simulink model "SUT_Test"  (Simulink 7.0)
settings: Solver=ode4  SolverMode=SingleTasking  StartTime=0.0  StopTime=252  FixedStep=0.01  RelTol=1e-3
InitFcn:
  | tempomat_para
StopFcn:
  | clear;
values from neighbouring files (symbols this model uses):
  A = 1.9    [tempomat_para.m]
  a_Fzg_max = 2    [tempomat_para.m]
  a_Fzg_min = -2    [tempomat_para.m]
  cw = 0.32    [tempomat_para.m]
  gang = [1 2 3 4]    [tempomat_para.m]
  gang_vec = [1 2 3 4]    [tempomat_para.m]
  i_anteil = 5    [tempomat_para.m]
  i_d = 3.42    [tempomat_para.m]
  i_g = [3.91 2.17 1.37 1.00]    [tempomat_para.m]
  lambda_gang = [1.3 1.25  1.17  1.05]    [tempomat_para.m]
  m_Fzg = 1400    [tempomat_para.m]
  M_mot_max = [130 149 163 170 168 166 162 158 150 139 123 80]    [tempomat_para.m]
  M_mot_min = [0 -40]    [tempomat_para.m]
  n_mot0 = 1000    [tempomat_para.m]
  n_mot_max = 1000:500:6500    [tempomat_para.m]
  n_mot_min = [1000 6500]    [tempomat_para.m]
  p_anteil = 100    [tempomat_para.m]
  r_dyn = 0.28    [tempomat_para.m]
  rho = 1.202    [tempomat_para.m]
  t_sch = 0.2    [tempomat_para.m]
  TI = [block '/TI']    [PSTI_callback.m]
  v_Fzg_ms0 = 0    [tempomat_para.m]
undefined symbols (not defined in the file or in its folder): Drossel_mat, getdatatypespecs
libraries: simulink x116, fzgbib x6
(part 10 of 11)

== system SUT_Test/Test Specification/R1 Speed Control step response/Maximum overshoot < 5 &  Steady state error < 5/Step response characteristics/Step response trigger/Active if signals constant for some specified time/Time since signal constant1 ==
  Signal : Inport  OutDataType=sfix(16)  OutScaling=2^0
  Clock : Clock
      settings: Decimation=10
  Detect constant : Subsystem  TreatAsAtomicUnit=on  mask(Feature extraction block){RT=0.0001}
      mask prompts: RT "Relative tolerance in %"
      mask help: Detect if the signal value is constant (using the last two signal values) allowing for a user-defined relative deviation
      mask CallbackString:
      | if or( (str2double(get_param(gcb,'RT')) < 0), (str2double(get_param(gcb,'RT')) > 100))
      |     error(['Relative tolerance value (' get_param(gcb,'RT') ') out of range. Please give a value between 0 and 100.']);
      | else
      |     set_param([gcb '/Relative tolerance/Relative Tolerance'],'Value',get_param(gcb,'RT'));
      | end
  Logical Operator : Logic  Operator=NAND  AllPortsSameDT=off  OutDataTypeMode=boolean
  Logical Operator1 : Logic  Operator=NOT  AllPortsSameDT=off  OutDataTypeMode=boolean
  Memory : Memory  Orientation=left
  Memory1 : Memory
  Subtract : Sum  Inputs=-+  OutDataType=sfix(16)  OutScaling=2^-10
  Switch : Switch  Criteria=u2 > Threshold
  Trigger : Outport  OutDataType=sfix(16)  OutScaling=2^0
  Feature : Outport  Port=2  OutDataType=sfix(16)  OutScaling=2^0
  wires:
  Logical Operator/1 -> Switch/2
  Logical Operator1/1 -> Logical Operator/2
  Memory1/1 -> Logical Operator1/1
  Memory/1 -> Switch/1
  Switch/1 -> Memory/1, Subtract/1
  Clock/1 -> Switch/3, Subtract/2
  Subtract/1 -> Feature/1
  Detect constant/1(Constant) -> Memory1/1, Logical Operator/1, Trigger/1
  Signal/1 -> Detect constant/1(Signal)

== system SUT_Test/Test Specification/R2 Speed Control velocity restoration time after simple  acceleration/deceleration/CC active + no target & Speed Control active & step of V_Des = |1|  with time periods >= 7s/Step with step size=|1|  and time periods >= 6s detection/Step detection/Active if signals constant for some specified time/Time since signal constant1 ==
  Signal : Inport  OutDataType=sfix(16)  OutScaling=2^0
  Clock : Clock
      settings: Decimation=10
  Detect constant : Subsystem  TreatAsAtomicUnit=on  mask(Feature extraction block){RT=0.0001}
      mask prompts: RT "Relative tolerance in %"
      mask help: Detect if the signal value is constant (using the last two signal values) allowing for a user-defined relative deviation
      mask CallbackString:
      | if or( (str2double(get_param(gcb,'RT')) < 0), (str2double(get_param(gcb,'RT')) > 100))
      |     error(['Relative tolerance value (' get_param(gcb,'RT') ') out of range. Please give a value between 0 and 100.']);
      | else
      |     set_param([gcb '/Relative tolerance/Relative Tolerance'],'Value',get_param(gcb,'RT'));
      | end
  Logical Operator : Logic  Operator=NAND  AllPortsSameDT=off  OutDataTypeMode=boolean
  Logical Operator1 : Logic  Operator=NOT  AllPortsSameDT=off  OutDataTypeMode=boolean
  Memory : Memory  Orientation=left
  Memory1 : Memory
  Subtract : Sum  Inputs=-+  OutDataType=sfix(16)  OutScaling=2^-10
  Switch : Switch  Criteria=u2 > Threshold
  Trigger : Outport  OutDataType=sfix(16)  OutScaling=2^0
  Feature : Outport  Port=2  OutDataType=sfix(16)  OutScaling=2^0
  wires:
  Logical Operator/1 -> Switch/2
  Logical Operator1/1 -> Logical Operator/2
  Memory1/1 -> Logical Operator1/1
  Memory/1 -> Switch/1
  Switch/1 -> Memory/1, Subtract/1
  Clock/1 -> Switch/3, Subtract/2
  Subtract/1 -> Feature/1
  Detect constant/1(Constant) -> Memory1/1, Logical Operator/1, Trigger/1
  Signal/1 -> Detect constant/1(Signal)

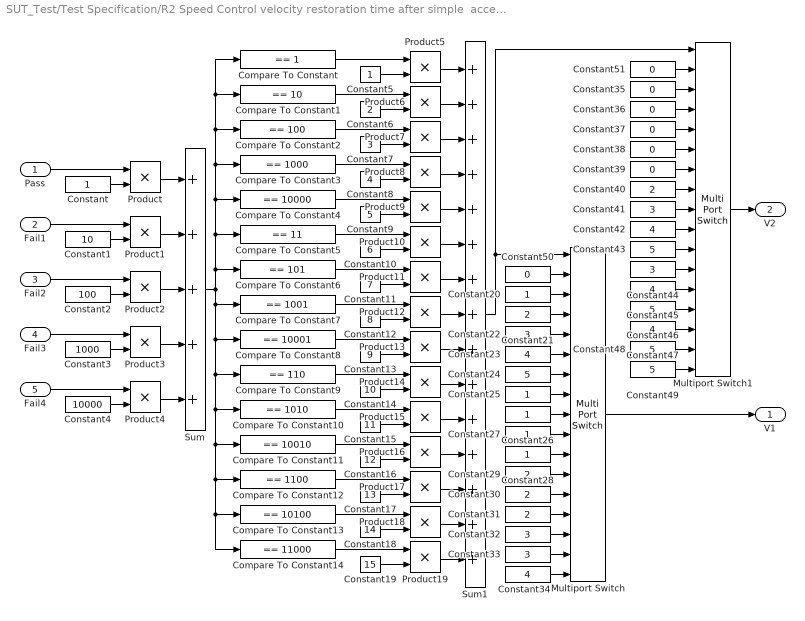
== system SUT_Test/Test Specification/R2 Speed Control velocity restoration time after simple  acceleration/deceleration/after (6 seconds)  |V_Des-V_Vhcl <= 1.4|/PAS1/none - pass - fail/Arbitration/Verdict identification ==
  Pass : Inport  OutDataType=sfix(16)  OutScaling=2^0
  Fail1 : Inport  Port=2  OutDataType=sfix(16)  OutScaling=2^0
  Fail2 : Inport  Port=3  OutDataType=sfix(16)  OutScaling=2^0
  Fail3 : Inport  Port=4  OutDataType=sfix(16)  OutScaling=2^0
  Fail4 : Inport  Port=5  OutDataType=sfix(16)  OutScaling=2^0
  Compare To Constant : simulink/Logic and Bit Operations/Compare To Constant  SystemSampleTime=-1  relop===  const=1  LogicOutDataTypeMode=uint8  ZeroCross=off
  Compare To Constant1 : simulink/Logic and Bit Operations/Compare To Constant  SystemSampleTime=-1  relop===  const=10  LogicOutDataTypeMode=uint8  ZeroCross=off
  Compare To Constant10 : simulink/Logic and Bit Operations/Compare To Constant  SystemSampleTime=-1  relop===  const=1010  LogicOutDataTypeMode=uint8  ZeroCross=off
  Compare To Constant11 : simulink/Logic and Bit Operations/Compare To Constant  SystemSampleTime=-1  relop===  const=10010  LogicOutDataTypeMode=uint8  ZeroCross=off
  Compare To Constant12 : simulink/Logic and Bit Operations/Compare To Constant  SystemSampleTime=-1  relop===  const=1100  LogicOutDataTypeMode=uint8  ZeroCross=off
  Compare To Constant13 : simulink/Logic and Bit Operations/Compare To Constant  SystemSampleTime=-1  relop===  const=10100  LogicOutDataTypeMode=uint8  ZeroCross=off
  Compare To Constant14 : simulink/Logic and Bit Operations/Compare To Constant  SystemSampleTime=-1  relop===  const=11000  LogicOutDataTypeMode=uint8  ZeroCross=off
  Compare To Constant2 : simulink/Logic and Bit Operations/Compare To Constant  SystemSampleTime=-1  relop===  const=100  LogicOutDataTypeMode=uint8  ZeroCross=off
  Compare To Constant3 : simulink/Logic and Bit Operations/Compare To Constant  SystemSampleTime=-1  relop===  const=1000  LogicOutDataTypeMode=uint8  ZeroCross=off
  Compare To Constant4 : simulink/Logic and Bit Operations/Compare To Constant  SystemSampleTime=-1  relop===  const=10000  LogicOutDataTypeMode=uint8  ZeroCross=off
  Compare To Constant5 : simulink/Logic and Bit Operations/Compare To Constant  SystemSampleTime=-1  relop===  const=11  LogicOutDataTypeMode=uint8  ZeroCross=off
  Compare To Constant6 : simulink/Logic and Bit Operations/Compare To Constant  SystemSampleTime=-1  relop===  const=101  LogicOutDataTypeMode=uint8  ZeroCross=off
  Compare To Constant7 : simulink/Logic and Bit Operations/Compare To Constant  SystemSampleTime=-1  relop===  const=1001  LogicOutDataTypeMode=uint8  ZeroCross=off
  Compare To Constant8 : simulink/Logic and Bit Operations/Compare To Constant  SystemSampleTime=-1  relop===  const=10001  LogicOutDataTypeMode=uint8  ZeroCross=off
  Compare To Constant9 : simulink/Logic and Bit Operations/Compare To Constant  SystemSampleTime=-1  relop===  const=110  LogicOutDataTypeMode=uint8  ZeroCross=off
  Constant{,5,20,25..28} (7 alike) : Constant  OutDataType=sfix(16)  OutScaling=2^0
  Constant1 : Constant  Value=10  OutDataType=sfix(16)  OutScaling=2^0
  Constant10 : Constant  Value=6  OutDataType=sfix(16)  OutScaling=2^0
  Constant11 : Constant  Value=7  OutDataType=sfix(16)  OutScaling=2^0
  Constant12 : Constant  Value=8  OutDataType=sfix(16)  OutScaling=2^0
  Constant13 : Constant  Value=9  OutDataType=sfix(16)  OutScaling=2^0
  Constant14 : Constant  Value=10  OutDataType=sfix(16)  OutScaling=2^0
  Constant15 : Constant  Value=11  OutDataType=sfix(16)  OutScaling=2^0
  Constant16 : Constant  Value=12  OutDataType=sfix(16)  OutScaling=2^0
  Constant17 : Constant  Value=13  OutDataType=sfix(16)  OutScaling=2^0
  Constant18 : Constant  Value=14  OutDataType=sfix(16)  OutScaling=2^0
  Constant19 : Constant  Value=15  OutDataType=sfix(16)  OutScaling=2^0
  Constant2 : Constant  Value=100  OutDataType=sfix(16)  OutScaling=2^0
  Constant{6,21,29..31,40} (6 alike) : Constant  Value=2  OutDataType=sfix(16)  OutScaling=2^0
  Constant{7,22,32..33,41,44} (6 alike) : Constant  Value=3  OutDataType=sfix(16)  OutScaling=2^0
  Constant{8,23,34,42,45,47} (6 alike) : Constant  Value=4  OutDataType=sfix(16)  OutScaling=2^0
  Constant{9,24,43,46,48..49} (6 alike) : Constant  Value=5  OutDataType=sfix(16)  OutScaling=2^0
  Constant3 : Constant  Value=1000  OutDataType=sfix(16)  OutScaling=2^0
  Constant{35..39,50..51} (7 alike) : Constant  Value=0  OutDataType=sfix(16)  OutScaling=2^0
  Constant4 : Constant  Value=10000  OutDataType=sfix(16)  OutScaling=2^0
  Multiport Switch : MultiPortSwitch  Inputs=16  zeroidx=on
  Multiport Switch1 : MultiPortSwitch  Inputs=16  zeroidx=on
  Product{,1..19} (20 alike) : Product  OutDataType=sfix(16)  OutScaling=2^0  RndMeth=Zero
  Sum : Sum  Inputs=+++++  OutDataType=sfix(16)  OutScaling=2^0
  Sum1 : Sum  Inputs=+++++++++++++++  OutDataType=sfix(16)  OutScaling=2^0
  V1 : Outport  OutDataType=sfix(16)  OutScaling=2^0
  V2 : Outport  Port=2  OutDataType=sfix(16)  OutScaling=2^0
  wires:
  Constant51/1 -> Multiport Switch1/2
  Constant34/1 -> Multiport Switch/17
  Constant33/1 -> Multiport Switch/16
  Constant32/1 -> Multiport Switch/15
  Constant31/1 -> Multiport Switch/14
  Constant30/1 -> Multiport Switch/13
  Constant29/1 -> Multiport Switch/12
  Constant28/1 -> Multiport Switch/11
  Constant27/1 -> Multiport Switch/10
  Constant26/1 -> Multiport Switch/9
  Constant25/1 -> Multiport Switch/8
  Constant24/1 -> Multiport Switch/7
  Constant23/1 -> Multiport Switch/6
  Constant22/1 -> Multiport Switch/5
  Constant21/1 -> Multiport Switch/4
  Constant20/1 -> Multiport Switch/3
  Constant50/1 -> Multiport Switch/2
  Product19/1 -> Sum1/15
  Product18/1 -> Sum1/14
  Product17/1 -> Sum1/13
  Product16/1 -> Sum1/12
  Product15/1 -> Sum1/11
  Product14/1 -> Sum1/10
  Product13/1 -> Sum1/9
  Product12/1 -> Sum1/8
  Product11/1 -> Sum1/7
  Product10/1 -> Sum1/6
  Product9/1 -> Sum1/5
  Product8/1 -> Sum1/4
  Product7/1 -> Sum1/3
  Product6/1 -> Sum1/2
  Product5/1 -> Sum1/1
  Multiport Switch1/1 -> V2/1
  Constant49/1 -> Multiport Switch1/17
  Constant48/1 -> Multiport Switch1/16
  Constant47/1 -> Multiport Switch1/15
  Constant46/1 -> Multiport Switch1/14
  Constant45/1 -> Multiport Switch1/13
  Constant44/1 -> Multiport Switch1/12
  Constant43/1 -> Multiport Switch1/11
  Constant42/1 -> Multiport Switch1/10
  Constant41/1 -> Multiport Switch1/9
  Constant40/1 -> Multiport Switch1/8
  Constant39/1 -> Multiport Switch1/7
  Constant38/1 -> Multiport Switch1/6
  Constant37/1 -> Multiport Switch1/5
  Constant36/1 -> Multiport Switch1/4
  Constant35/1 -> Multiport Switch1/3
  Sum1/1 -> Multiport Switch1/1, Multiport Switch/1
  Multiport Switch/1 -> V1/1
  Sum/1 -> Compare To Constant7/1, Compare To Constant13/1, Compare To Constant14/1, Compare To Constant12/1, Compare To Constant11/1, Compare To Constant10/1, Compare To Constant9/1, Compare To Constant8/1, Compare To Constant/1, Compare To Constant1/1, Compare To Constant2/1, Compare To Constant3/1, Compare To Constant4/1, Compare To Constant5/1, Compare To Constant6/1
  Compare To Constant14/1 -> Product19/1
  Constant19/1 -> Product19/2
  Compare To Constant13/1 -> Product18/1
  Constant18/1 -> Product18/2
  Compare To Constant12/1 -> Product17/1
  Constant17/1 -> Product17/2
  Compare To Constant11/1 -> Product16/1
  Constant16/1 -> Product16/2
  Compare To Constant10/1 -> Product15/1
  Constant15/1 -> Product15/2
  Compare To Constant9/1 -> Product14/1
  Constant14/1 -> Product14/2
  Compare To Constant8/1 -> Product13/1
  Constant13/1 -> Product13/2
  Compare To Constant7/1 -> Product12/1
  Constant12/1 -> Product12/2
  Compare To Constant6/1 -> Product11/1
  Constant11/1 -> Product11/2
  Compare To Constant5/1 -> Product10/1
  Constant10/1 -> Product10/2
  Compare To Constant4/1 -> Product9/1
  Constant9/1 -> Product9/2
  Compare To Constant3/1 -> Product8/1
  Compare To Constant2/1 -> Product7/1
  Constant8/1 -> Product8/2
  Constant7/1 -> Product7/2
  Compare To Constant1/1 -> Product6/1
  Constant6/1 -> Product6/2
  Constant5/1 -> Product5/2
  Compare To Constant/1 -> Product5/1
  Product4/1 -> Sum/5
  Product3/1 -> Sum/4
  Product2/1 -> Sum/3
  Product1/1 -> Sum/2
  Product/1 -> Sum/1
  Constant/1 -> Product/2
  Constant1/1 -> Product1/2
  Constant2/1 -> Product2/2
  Constant4/1 -> Product4/2
  Constant3/1 -> Product3/2
  Fail4/1 -> Product4/1
  Fail3/1 -> Product3/1
  Fail2/1 -> Product2/1
  Fail1/1 -> Product1/1
  Pass/1 -> Product/1

== system SUT_Test/Test Specification/R2 Speed Control velocity restoration time after simple  acceleration/deceleration/after (6 seconds)  |V_Des-V_Vhcl <= 1.4|/PAS1/none - pass - fail/Arbitration/Verdict selection ==
  V1 : Inport  OutDataType=sfix(16)  OutScaling=2^0
  V2 : Inport  Port=2  OutDataType=sfix(16)  OutScaling=2^0
  Delay P F1 F3 : Inport  Port=3  OutDataType=sfix(16)  OutScaling=2^0
  Delay F2 : Inport  Port=4  OutDataType=sfix(16)  OutScaling=2^0
  Delay F4 : Inport  Port=5  OutDataType=sfix(16)  OutScaling=2^0
  Max delay : Inport  Port=6  OutDataType=sfix(16)  OutScaling=2^0
  Compare To Zero1 : simulink/Logic and Bit Operations/Compare To Zero  SystemSampleTime=-1  relop=~=  LogicOutDataTypeMode=boolean  ZeroCross=off
  Constant{2..4,39} (4 alike) : Constant  Value=0  OutDataType=sfix(16)  OutScaling=2^0
  Constant35 : Constant  OutDataType=sfix(16)  OutScaling=2^0
  Constant40 : Constant  Value=2  OutDataType=sfix(16)  OutScaling=2^0
  Memory : Memory
  Memory1 : Memory
  Multiport Switch1 : MultiPortSwitch  Inputs=6  zeroidx=on
  Multiport Switch2 : MultiPortSwitch  Inputs=6  zeroidx=on
  Multiport Switch4 : MultiPortSwitch  Inputs=6  zeroidx=on
  Sum : Sum  OutDataType=sfix(16)  OutScaling=2^0
  Switch : Switch  Criteria=u2 ~= 0
  Switch1 : Switch  Criteria=u2 ~= 0
  Switch2 : Switch  Criteria=u2 ~= 0
  Unit : Constant  OutDataType=sfix(16)  OutScaling=2^0
  Verdict : Outport  OutDataType=sfix(16)  OutScaling=2^0
  Delay : Outport  Port=2  OutDataType=sfix(16)  OutScaling=2^0
  wires:
  Switch2/1 -> Multiport Switch4/1, Memory/1
  Unit/1 -> Sum/1
  Memory1/1 -> Sum/2
  Sum/1 -> Switch1/1
  Multiport Switch4/1 -> Memory1/1
  Multiport Switch2/1 -> Switch1/3
  Switch1/1 -> Delay/1
  Switch/1 -> Multiport Switch1/1
  Compare To Zero1/1 -> Switch2/2, Switch1/2, Switch/2
  Memory/1 -> Switch/1, Compare To Zero1/1
  Delay F4/1 -> Multiport Switch4/7, Multiport Switch2/7
  Delay F2/1 -> Multiport Switch4/5, Multiport Switch2/5
  Delay P F1 F3/1 -> Multiport Switch4/3, Multiport Switch4/4, Multiport Switch4/6, Multiport Switch2/4, Multiport Switch2/6, Multiport Switch2/3
  Max delay/1 -> Multiport Switch4/2, Multiport Switch2/2
  V1/1 -> Switch2/1, Switch/3, Multiport Switch2/1
  V2/1 -> Switch2/3
  Constant40/1 -> Multiport Switch1/2
  Constant35/1 -> Multiport Switch1/3
  Constant4/1 -> Multiport Switch1/4
  Constant3/1 -> Multiport Switch1/5
  Constant2/1 -> Multiport Switch1/6
  Constant39/1 -> Multiport Switch1/7
  Multiport Switch1/1 -> Verdict/1

== system SUT_Test/Test Specification/R2 Speed Control velocity restoration time after simple  acceleration/deceleration/after (6 seconds)  |V_Des-V_Vhcl <= 1.4|/PAS1/none - pass - fail/Compute delay/Hold1 ==
  " " : Inport  OutDataType=sfix(16)  OutScaling=2^0
  "    " : Inport  Port=2  OutDataType=sfix(16)  OutScaling=2^0
  Memory : Memory  Orientation=left
  Switch : Switch  Criteria=u2 ~= 0
  "  " : Outport  OutDataType=sfix(16)  OutScaling=2^0
  wires:
  " "/1 -> Switch/2
  "    "/1 -> Switch/1
  Switch/1 -> "  "/1, Memory/1
  Memory/1 -> Switch/3

== system SUT_Test/Test Specification/R2 Speed Control velocity restoration time after simple  acceleration/deceleration/after (6 seconds)  |V_Des-V_Vhcl <= 1.4|/PAS1/none - pass - fail/Compute delay1/Hold1 ==
  " " : Inport  OutDataType=sfix(16)  OutScaling=2^0
  "    " : Inport  Port=2  OutDataType=sfix(16)  OutScaling=2^0
  Memory : Memory  Orientation=left
  Switch : Switch  Criteria=u2 ~= 0
  "  " : Outport  OutDataType=sfix(16)  OutScaling=2^0
  wires:
  " "/1 -> Switch/2
  "    "/1 -> Switch/1
  Switch/1 -> "  "/1, Memory/1
  Memory/1 -> Switch/3

== system SUT_Test/Test Specification/R2 Speed Control velocity restoration time after simple  acceleration/deceleration/after (6 seconds)  |V_Des-V_Vhcl <= 1.4|/PAS1/none - pass - fail/Compute delay2/Hold1 ==
  " " : Inport  OutDataType=sfix(16)  OutScaling=2^0
  "    " : Inport  Port=2  OutDataType=sfix(16)  OutScaling=2^0
  Memory : Memory  Orientation=left
  Switch : Switch  Criteria=u2 ~= 0
  "  " : Outport  OutDataType=sfix(16)  OutScaling=2^0
  wires:
  Memory/1 -> Switch/3
  Switch/1 -> Memory/1, "  "/1
  "    "/1 -> Switch/1
  " "/1 -> Switch/2

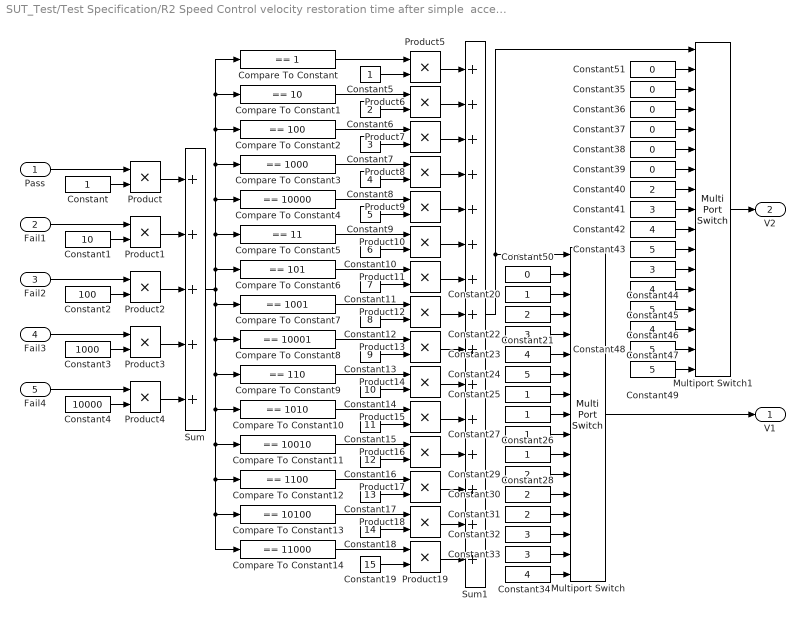
== system SUT_Test/Test Specification/R2 Speed Control velocity restoration time after simple  acceleration/deceleration/after (6 seconds)  |V_Des-V_Vhcl <= 1.4|/PAS2/none - pass - fail/Arbitration/Verdict identification ==
  Pass : Inport  OutDataType=sfix(16)  OutScaling=2^0
  Fail1 : Inport  Port=2  OutDataType=sfix(16)  OutScaling=2^0
  Fail2 : Inport  Port=3  OutDataType=sfix(16)  OutScaling=2^0
  Fail3 : Inport  Port=4  OutDataType=sfix(16)  OutScaling=2^0
  Fail4 : Inport  Port=5  OutDataType=sfix(16)  OutScaling=2^0
  Compare To Constant : simulink/Logic and Bit Operations/Compare To Constant  SystemSampleTime=-1  relop===  const=1  LogicOutDataTypeMode=uint8  ZeroCross=off
  Compare To Constant1 : simulink/Logic and Bit Operations/Compare To Constant  SystemSampleTime=-1  relop===  const=10  LogicOutDataTypeMode=uint8  ZeroCross=off
  Compare To Constant10 : simulink/Logic and Bit Operations/Compare To Constant  SystemSampleTime=-1  relop===  const=1010  LogicOutDataTypeMode=uint8  ZeroCross=off
  Compare To Constant11 : simulink/Logic and Bit Operations/Compare To Constant  SystemSampleTime=-1  relop===  const=10010  LogicOutDataTypeMode=uint8  ZeroCross=off
  Compare To Constant12 : simulink/Logic and Bit Operations/Compare To Constant  SystemSampleTime=-1  relop===  const=1100  LogicOutDataTypeMode=uint8  ZeroCross=off
  Compare To Constant13 : simulink/Logic and Bit Operations/Compare To Constant  SystemSampleTime=-1  relop===  const=10100  LogicOutDataTypeMode=uint8  ZeroCross=off
  Compare To Constant14 : simulink/Logic and Bit Operations/Compare To Constant  SystemSampleTime=-1  relop===  const=11000  LogicOutDataTypeMode=uint8  ZeroCross=off
  Compare To Constant2 : simulink/Logic and Bit Operations/Compare To Constant  SystemSampleTime=-1  relop===  const=100  LogicOutDataTypeMode=uint8  ZeroCross=off
  Compare To Constant3 : simulink/Logic and Bit Operations/Compare To Constant  SystemSampleTime=-1  relop===  const=1000  LogicOutDataTypeMode=uint8  ZeroCross=off
  Compare To Constant4 : simulink/Logic and Bit Operations/Compare To Constant  SystemSampleTime=-1  relop===  const=10000  LogicOutDataTypeMode=uint8  ZeroCross=off
  Compare To Constant5 : simulink/Logic and Bit Operations/Compare To Constant  SystemSampleTime=-1  relop===  const=11  LogicOutDataTypeMode=uint8  ZeroCross=off
  Compare To Constant6 : simulink/Logic and Bit Operations/Compare To Constant  SystemSampleTime=-1  relop===  const=101  LogicOutDataTypeMode=uint8  ZeroCross=off
  Compare To Constant7 : simulink/Logic and Bit Operations/Compare To Constant  SystemSampleTime=-1  relop===  const=1001  LogicOutDataTypeMode=uint8  ZeroCross=off
  Compare To Constant8 : simulink/Logic and Bit Operations/Compare To Constant  SystemSampleTime=-1  relop===  const=10001  LogicOutDataTypeMode=uint8  ZeroCross=off
  Compare To Constant9 : simulink/Logic and Bit Operations/Compare To Constant  SystemSampleTime=-1  relop===  const=110  LogicOutDataTypeMode=uint8  ZeroCross=off
  Constant{,5,20,25..28} (7 alike) : Constant  OutDataType=sfix(16)  OutScaling=2^0
  Constant1 : Constant  Value=10  OutDataType=sfix(16)  OutScaling=2^0
  Constant10 : Constant  Value=6  OutDataType=sfix(16)  OutScaling=2^0
  Constant11 : Constant  Value=7  OutDataType=sfix(16)  OutScaling=2^0
  Constant12 : Constant  Value=8  OutDataType=sfix(16)  OutScaling=2^0
  Constant13 : Constant  Value=9  OutDataType=sfix(16)  OutScaling=2^0
  Constant14 : Constant  Value=10  OutDataType=sfix(16)  OutScaling=2^0
  Constant15 : Constant  Value=11  OutDataType=sfix(16)  OutScaling=2^0
  Constant16 : Constant  Value=12  OutDataType=sfix(16)  OutScaling=2^0
  Constant17 : Constant  Value=13  OutDataType=sfix(16)  OutScaling=2^0
  Constant18 : Constant  Value=14  OutDataType=sfix(16)  OutScaling=2^0
  Constant19 : Constant  Value=15  OutDataType=sfix(16)  OutScaling=2^0
  Constant2 : Constant  Value=100  OutDataType=sfix(16)  OutScaling=2^0
  Constant{6,21,29..31,40} (6 alike) : Constant  Value=2  OutDataType=sfix(16)  OutScaling=2^0
  Constant{7,22,32..33,41,44} (6 alike) : Constant  Value=3  OutDataType=sfix(16)  OutScaling=2^0
  Constant{8,23,34,42,45,47} (6 alike) : Constant  Value=4  OutDataType=sfix(16)  OutScaling=2^0
  Constant{9,24,43,46,48..49} (6 alike) : Constant  Value=5  OutDataType=sfix(16)  OutScaling=2^0
  Constant3 : Constant  Value=1000  OutDataType=sfix(16)  OutScaling=2^0
  Constant{35..39,50..51} (7 alike) : Constant  Value=0  OutDataType=sfix(16)  OutScaling=2^0
  Constant4 : Constant  Value=10000  OutDataType=sfix(16)  OutScaling=2^0
  Multiport Switch : MultiPortSwitch  Inputs=16  zeroidx=on
  Multiport Switch1 : MultiPortSwitch  Inputs=16  zeroidx=on
  Product{,1..19} (20 alike) : Product  OutDataType=sfix(16)  OutScaling=2^0  RndMeth=Zero
  Sum : Sum  Inputs=+++++  OutDataType=sfix(16)  OutScaling=2^0
  Sum1 : Sum  Inputs=+++++++++++++++  OutDataType=sfix(16)  OutScaling=2^0
  V1 : Outport  OutDataType=sfix(16)  OutScaling=2^0
  V2 : Outport  Port=2  OutDataType=sfix(16)  OutScaling=2^0
  wires:
  Constant51/1 -> Multiport Switch1/2
  Constant34/1 -> Multiport Switch/17
  Constant33/1 -> Multiport Switch/16
  Constant32/1 -> Multiport Switch/15
  Constant31/1 -> Multiport Switch/14
  Constant30/1 -> Multiport Switch/13
  Constant29/1 -> Multiport Switch/12
  Constant28/1 -> Multiport Switch/11
  Constant27/1 -> Multiport Switch/10
  Constant26/1 -> Multiport Switch/9
  Constant25/1 -> Multiport Switch/8
  Constant24/1 -> Multiport Switch/7
  Constant23/1 -> Multiport Switch/6
  Constant22/1 -> Multiport Switch/5
  Constant21/1 -> Multiport Switch/4
  Constant20/1 -> Multiport Switch/3
  Constant50/1 -> Multiport Switch/2
  Product19/1 -> Sum1/15
  Product18/1 -> Sum1/14
  Product17/1 -> Sum1/13
  Product16/1 -> Sum1/12
  Product15/1 -> Sum1/11
  Product14/1 -> Sum1/10
  Product13/1 -> Sum1/9
  Product12/1 -> Sum1/8
  Product11/1 -> Sum1/7
  Product10/1 -> Sum1/6
  Product9/1 -> Sum1/5
  Product8/1 -> Sum1/4
  Product7/1 -> Sum1/3
  Product6/1 -> Sum1/2
  Product5/1 -> Sum1/1
  Multiport Switch1/1 -> V2/1
  Constant49/1 -> Multiport Switch1/17
  Constant48/1 -> Multiport Switch1/16
  Constant47/1 -> Multiport Switch1/15
  Constant46/1 -> Multiport Switch1/14
  Constant45/1 -> Multiport Switch1/13
  Constant44/1 -> Multiport Switch1/12
  Constant43/1 -> Multiport Switch1/11
  Constant42/1 -> Multiport Switch1/10
  Constant41/1 -> Multiport Switch1/9
  Constant40/1 -> Multiport Switch1/8
  Constant39/1 -> Multiport Switch1/7
  Constant38/1 -> Multiport Switch1/6
  Constant37/1 -> Multiport Switch1/5
  Constant36/1 -> Multiport Switch1/4
  Constant35/1 -> Multiport Switch1/3
  Sum1/1 -> Multiport Switch1/1, Multiport Switch/1
  Multiport Switch/1 -> V1/1
  Sum/1 -> Compare To Constant7/1, Compare To Constant13/1, Compare To Constant14/1, Compare To Constant12/1, Compare To Constant11/1, Compare To Constant10/1, Compare To Constant9/1, Compare To Constant8/1, Compare To Constant/1, Compare To Constant1/1, Compare To Constant2/1, Compare To Constant3/1, Compare To Constant4/1, Compare To Constant5/1, Compare To Constant6/1
  Compare To Constant14/1 -> Product19/1
  Constant19/1 -> Product19/2
  Compare To Constant13/1 -> Product18/1
  Constant18/1 -> Product18/2
  Compare To Constant12/1 -> Product17/1
  Constant17/1 -> Product17/2
  Compare To Constant11/1 -> Product16/1
  Constant16/1 -> Product16/2
  Compare To Constant10/1 -> Product15/1
  Constant15/1 -> Product15/2
  Compare To Constant9/1 -> Product14/1
  Constant14/1 -> Product14/2
  Compare To Constant8/1 -> Product13/1
  Constant13/1 -> Product13/2
  Compare To Constant7/1 -> Product12/1
  Constant12/1 -> Product12/2
  Compare To Constant6/1 -> Product11/1
  Constant11/1 -> Product11/2
  Compare To Constant5/1 -> Product10/1
  Constant10/1 -> Product10/2
  Compare To Constant4/1 -> Product9/1
  Constant9/1 -> Product9/2
  Compare To Constant3/1 -> Product8/1
  Compare To Constant2/1 -> Product7/1
  Constant8/1 -> Product8/2
  Constant7/1 -> Product7/2
  Compare To Constant1/1 -> Product6/1
  Constant6/1 -> Product6/2
  Constant5/1 -> Product5/2
  Compare To Constant/1 -> Product5/1
  Product4/1 -> Sum/5
  Product3/1 -> Sum/4
  Product2/1 -> Sum/3
  Product1/1 -> Sum/2
  Product/1 -> Sum/1
  Constant/1 -> Product/2
  Constant1/1 -> Product1/2
  Constant2/1 -> Product2/2
  Constant4/1 -> Product4/2
  Constant3/1 -> Product3/2
  Fail4/1 -> Product4/1
  Fail3/1 -> Product3/1
  Fail2/1 -> Product2/1
  Fail1/1 -> Product1/1
  Pass/1 -> Product/1

== system SUT_Test/Test Specification/R2 Speed Control velocity restoration time after simple  acceleration/deceleration/after (6 seconds)  |V_Des-V_Vhcl <= 1.4|/PAS2/none - pass - fail/Arbitration/Verdict selection ==
  V1 : Inport  OutDataType=sfix(16)  OutScaling=2^0
  V2 : Inport  Port=2  OutDataType=sfix(16)  OutScaling=2^0
  Delay P F1 F3 : Inport  Port=3  OutDataType=sfix(16)  OutScaling=2^0
  Delay F2 : Inport  Port=4  OutDataType=sfix(16)  OutScaling=2^0
  Delay F4 : Inport  Port=5  OutDataType=sfix(16)  OutScaling=2^0
  Max delay : Inport  Port=6  OutDataType=sfix(16)  OutScaling=2^0
  Compare To Zero1 : simulink/Logic and Bit Operations/Compare To Zero  SystemSampleTime=-1  relop=~=  LogicOutDataTypeMode=boolean  ZeroCross=off
  Constant{2..4,39} (4 alike) : Constant  Value=0  OutDataType=sfix(16)  OutScaling=2^0
  Constant35 : Constant  OutDataType=sfix(16)  OutScaling=2^0
  Constant40 : Constant  Value=2  OutDataType=sfix(16)  OutScaling=2^0
  Memory : Memory
  Memory1 : Memory
  Multiport Switch1 : MultiPortSwitch  Inputs=6  zeroidx=on
  Multiport Switch2 : MultiPortSwitch  Inputs=6  zeroidx=on
  Multiport Switch4 : MultiPortSwitch  Inputs=6  zeroidx=on
  Sum : Sum  OutDataType=sfix(16)  OutScaling=2^0
  Switch : Switch  Criteria=u2 ~= 0
  Switch1 : Switch  Criteria=u2 ~= 0
  Switch2 : Switch  Criteria=u2 ~= 0
  Unit : Constant  OutDataType=sfix(16)  OutScaling=2^0
  Verdict : Outport  OutDataType=sfix(16)  OutScaling=2^0
  Delay : Outport  Port=2  OutDataType=sfix(16)  OutScaling=2^0
  wires:
  Switch2/1 -> Multiport Switch4/1, Memory/1
  Unit/1 -> Sum/1
  Memory1/1 -> Sum/2
  Sum/1 -> Switch1/1
  Multiport Switch4/1 -> Memory1/1
  Multiport Switch2/1 -> Switch1/3
  Switch1/1 -> Delay/1
  Switch/1 -> Multiport Switch1/1
  Compare To Zero1/1 -> Switch2/2, Switch1/2, Switch/2
  Memory/1 -> Switch/1, Compare To Zero1/1
  Delay F4/1 -> Multiport Switch4/7, Multiport Switch2/7
  Delay F2/1 -> Multiport Switch4/5, Multiport Switch2/5
  Delay P F1 F3/1 -> Multiport Switch4/3, Multiport Switch4/4, Multiport Switch4/6, Multiport Switch2/4, Multiport Switch2/6, Multiport Switch2/3
  Max delay/1 -> Multiport Switch4/2, Multiport Switch2/2
  V1/1 -> Switch2/1, Switch/3, Multiport Switch2/1
  V2/1 -> Switch2/3
  Constant40/1 -> Multiport Switch1/2
  Constant35/1 -> Multiport Switch1/3
  Constant4/1 -> Multiport Switch1/4
  Constant3/1 -> Multiport Switch1/5
  Constant2/1 -> Multiport Switch1/6
  Constant39/1 -> Multiport Switch1/7
  Multiport Switch1/1 -> Verdict/1

== system SUT_Test/Test Specification/R2 Speed Control velocity restoration time after simple  acceleration/deceleration/after (6 seconds)  |V_Des-V_Vhcl <= 1.4|/PAS2/none - pass - fail/Compute delay/Hold1 ==
  " " : Inport  OutDataType=sfix(16)  OutScaling=2^0
  "    " : Inport  Port=2  OutDataType=sfix(16)  OutScaling=2^0
  Memory : Memory  Orientation=left
  Switch : Switch  Criteria=u2 ~= 0
  "  " : Outport  OutDataType=sfix(16)  OutScaling=2^0
  wires:
  " "/1 -> Switch/2
  "    "/1 -> Switch/1
  Switch/1 -> "  "/1, Memory/1
  Memory/1 -> Switch/3

== system SUT_Test/Test Specification/R2 Speed Control velocity restoration time after simple  acceleration/deceleration/after (6 seconds)  |V_Des-V_Vhcl <= 1.4|/PAS2/none - pass - fail/Compute delay1/Hold1 ==
  " " : Inport  OutDataType=sfix(16)  OutScaling=2^0
  "    " : Inport  Port=2  OutDataType=sfix(16)  OutScaling=2^0
  Memory : Memory  Orientation=left
  Switch : Switch  Criteria=u2 ~= 0
  "  " : Outport  OutDataType=sfix(16)  OutScaling=2^0
  wires:
  " "/1 -> Switch/2
  "    "/1 -> Switch/1
  Switch/1 -> "  "/1, Memory/1
  Memory/1 -> Switch/3

== system SUT_Test/Test Specification/R2 Speed Control velocity restoration time after simple  acceleration/deceleration/after (6 seconds)  |V_Des-V_Vhcl <= 1.4|/PAS2/none - pass - fail/Compute delay2/Hold1 ==
  " " : Inport  OutDataType=sfix(16)  OutScaling=2^0
  "    " : Inport  Port=2  OutDataType=sfix(16)  OutScaling=2^0
  Memory : Memory  Orientation=left
  Switch : Switch  Criteria=u2 ~= 0
  "  " : Outport  OutDataType=sfix(16)  OutScaling=2^0
  wires:
  Memory/1 -> Switch/3
  Switch/1 -> Memory/1, "  "/1
  "    "/1 -> Switch/1
  " "/1 -> Switch/2

== system SUT_Test/Test Specification/R2 Speed Control velocity restoration time after simple  acceleration/deceleration/after (6 seconds)  |V_Des-V_Vhcl <= 1.4|/R = 2/Active for  6s after R=1 /Time since R = 1/R = 1 ==
  In1 : Inport  OutDataType=sfix(16)  OutScaling=2^0
  Bus Selector1 : BusSelector  OutputSignals=R
  Constant : Constant  OutDataType=sfix(16)  OutScaling=2^0
  Relational Operator : RelationalOperator  Operator===  LogicOutDataTypeMode=boolean
  Out1 : Outport  OutDataType=sfix(16)  OutScaling=2^0
  wires:
  In1/1 -> Bus Selector1/1
  Constant/1 -> Relational Operator/2
  Bus Selector1/1 -> Relational Operator/1  "<R>"
  Relational Operator/1 -> Out1/1

== system SUT_Test/Test Specification/R1 Speed Control step response/Complete step & CC active + no target & Speed Control active/Complete step detection/Step detection/Active if signals constant for some specified time/Time since signal constant/Detect constant ==
  Signal : Inport  OutDataType=sfix(16)  OutScaling=2^0
  Clock : Clock
      settings: Decimation=10
  Constant1 : Constant  Value=0  OutDataTypeMode=boolean  OutDataType=sfix(16)  OutScaling=2^0
  Memory : Memory
  Relative tolerance : Subsystem
  Switch : Switch  Criteria=u2 > Threshold
  Constant : Outport  OutDataType=sfix(16)  OutScaling=2^0
  wires:
  Switch/1 -> Constant/1
  Relative tolerance/1(sig == ref) -> Switch/1
  Clock/1 -> Switch/2
  Constant1/1 -> Switch/3
  Memory/1 -> Relative tolerance/2(ref)
  Signal/1 -> Relative tolerance/1(sig), Memory/1

== system SUT_Test/Test Specification/R1 Speed Control step response/Complete step & CC active + no target & Speed Control active/Complete step detection/Step detection/Active if signals constant for some specified time/Time since signal constant1/Detect constant ==
  Signal : Inport  OutDataType=sfix(16)  OutScaling=2^0
  Clock : Clock
      settings: Decimation=10
  Constant1 : Constant  Value=0  OutDataTypeMode=boolean  OutDataType=sfix(16)  OutScaling=2^0
  Memory : Memory
  Relative tolerance : Subsystem
  Switch : Switch  Criteria=u2 > Threshold
  Constant : Outport  OutDataType=sfix(16)  OutScaling=2^0
  wires:
  Signal/1 -> Relative tolerance/1(sig), Memory/1
  Memory/1 -> Relative tolerance/2(ref)
  Constant1/1 -> Switch/3
  Clock/1 -> Switch/2
  Relative tolerance/1(sig == ref) -> Switch/1
  Switch/1 -> Constant/1

== system SUT_Test/Test Specification/R1 Speed Control step response/Complete step & CC active + no target & Speed Control active/Complete step detection/Step detection reset/Active if signals constant for some specified time/Time since signal constant/Detect constant ==
  Signal : Inport  OutDataType=sfix(16)  OutScaling=2^0
  Clock : Clock
      settings: Decimation=10
  Constant1 : Constant  Value=0  OutDataTypeMode=boolean  OutDataType=sfix(16)  OutScaling=2^0
  Memory : Memory
  Relative tolerance : Subsystem
  Switch : Switch  Criteria=u2 > Threshold
  Constant : Outport  OutDataType=sfix(16)  OutScaling=2^0
  wires:
  Signal/1 -> Memory/1, Relative tolerance/1(sig)
  Memory/1 -> Relative tolerance/2(ref)
  Constant1/1 -> Switch/3
  Clock/1 -> Switch/2
  Relative tolerance/1(sig == ref) -> Switch/1
  Switch/1 -> Constant/1

== system SUT_Test/Test Specification/R1 Speed Control step response/Complete step & CC active + no target & Speed Control active/Complete step detection/Step detection reset/Active if signals constant for some specified time/Time since signal constant1/Detect constant ==
  Signal : Inport  OutDataType=sfix(16)  OutScaling=2^0
  Clock : Clock
      settings: Decimation=10
  Constant1 : Constant  Value=0  OutDataTypeMode=boolean  OutDataType=sfix(16)  OutScaling=2^0
  Memory : Memory
  Relative tolerance : Subsystem
  Switch : Switch  Criteria=u2 > Threshold
  Constant : Outport  OutDataType=sfix(16)  OutScaling=2^0
  wires:
  Switch/1 -> Constant/1
  Relative tolerance/1(sig == ref) -> Switch/1
  Clock/1 -> Switch/2
  Constant1/1 -> Switch/3
  Memory/1 -> Relative tolerance/2(ref)
  Signal/1 -> Memory/1, Relative tolerance/1(sig)

== system SUT_Test/Test Specification/R1 Speed Control step response/Maximum overshoot < 5 &  Steady state error < 5/Step response characteristics/Step response characteristics extraction/Extract maximum overshoot/Active if signals constant for some specified time/Time since signal constant ==
  Signal : Inport  OutDataType=sfix(16)  OutScaling=2^0
  Clock : Clock
      settings: Decimation=10
  Detect constant : Subsystem  TreatAsAtomicUnit=on  mask(Feature extraction block){RT=0.0001}
      mask prompts: RT "Relative tolerance in %"
      mask help: Detect if the signal value is constant (using the last two signal values) allowing for a user-defined relative deviation
      mask CallbackString:
      | if or( (str2double(get_param(gcb,'RT')) < 0), (str2double(get_param(gcb,'RT')) > 100))
      |     error(['Relative tolerance value (' get_param(gcb,'RT') ') out of range. Please give a value between 0 and 100.']);
      | else
      |     set_param([gcb '/Relative tolerance/Relative Tolerance'],'Value',get_param(gcb,'RT'));
      | end
  Logical Operator : Logic  Operator=NAND  AllPortsSameDT=off  OutDataTypeMode=boolean
  Logical Operator1 : Logic  Operator=NOT  AllPortsSameDT=off  OutDataTypeMode=boolean
  Memory : Memory  Orientation=left
  Memory1 : Memory
  Subtract : Sum  Inputs=-+  OutDataType=sfix(16)  OutScaling=2^-10
  Switch : Switch  Criteria=u2 > Threshold
  Trigger : Outport  OutDataType=sfix(16)  OutScaling=2^0
  Feature : Outport  Port=2  OutDataType=sfix(16)  OutScaling=2^0
  wires:
  Signal/1 -> Detect constant/1(Signal)
  Detect constant/1(Constant) -> Trigger/1, Logical Operator/1, Memory1/1
  Subtract/1 -> Feature/1
  Clock/1 -> Subtract/2, Switch/3
  Switch/1 -> Subtract/1, Memory/1
  Memory/1 -> Switch/1
  Memory1/1 -> Logical Operator1/1
  Logical Operator1/1 -> Logical Operator/2
  Logical Operator/1 -> Switch/2

== system SUT_Test/Test Specification/R1 Speed Control step response/Maximum overshoot < 5 &  Steady state error < 5/Step response characteristics/Step response characteristics extraction/Extract maximum overshoot/Active if signals constant for some specified time/Time since signal constant1 ==
  Signal : Inport  OutDataType=sfix(16)  OutScaling=2^0
  Clock : Clock
      settings: Decimation=10
  Detect constant : Subsystem  TreatAsAtomicUnit=on  mask(Feature extraction block){RT=0.0001}
      mask prompts: RT "Relative tolerance in %"
      mask help: Detect if the signal value is constant (using the last two signal values) allowing for a user-defined relative deviation
      mask CallbackString:
      | if or( (str2double(get_param(gcb,'RT')) < 0), (str2double(get_param(gcb,'RT')) > 100))
      |     error(['Relative tolerance value (' get_param(gcb,'RT') ') out of range. Please give a value between 0 and 100.']);
      | else
      |     set_param([gcb '/Relative tolerance/Relative Tolerance'],'Value',get_param(gcb,'RT'));
      | end
  Logical Operator : Logic  Operator=NAND  AllPortsSameDT=off  OutDataTypeMode=boolean
  Logical Operator1 : Logic  Operator=NOT  AllPortsSameDT=off  OutDataTypeMode=boolean
  Memory : Memory  Orientation=left
  Memory1 : Memory
  Subtract : Sum  Inputs=-+  OutDataType=sfix(16)  OutScaling=2^-10
  Switch : Switch  Criteria=u2 > Threshold
  Trigger : Outport  OutDataType=sfix(16)  OutScaling=2^0
  Feature : Outport  Port=2  OutDataType=sfix(16)  OutScaling=2^0
  wires:
  Logical Operator/1 -> Switch/2
  Logical Operator1/1 -> Logical Operator/2
  Memory1/1 -> Logical Operator1/1
  Memory/1 -> Switch/1
  Switch/1 -> Memory/1, Subtract/1
  Clock/1 -> Switch/3, Subtract/2
  Subtract/1 -> Feature/1
  Detect constant/1(Constant) -> Memory1/1, Logical Operator/1, Trigger/1
  Signal/1 -> Detect constant/1(Signal)

== system SUT_Test/Test Specification/R1 Speed Control step response/Maximum overshoot < 5 &  Steady state error < 5/Step response characteristics/Step response characteristics extraction/Extract maximum overshoot/Hold value with counter/Execution counter ==
  Reset : Inport  OutDataType=sfix(16)  OutScaling=2^0
  Add1 : Sum  OutDataType=sfix(16)  OutScaling=2^-10
  Constant : Constant  OutDataType=sfix(16)  OutScaling=2^0
  Logical Operator : Logic  Operator=NOT  AllPortsSameDT=off  OutDataTypeMode=Specify via dialog
  Memory : Memory  Orientation=left  InheritSampleTime=on
  Product : Product  OutDataType=sfix(16)  OutScaling=2^0  RndMeth=Zero
  Counter : Outport  OutDataType=sfix(16)  OutScaling=2^0
  wires:
  Product/1 -> Counter/1, Memory/1
  Logical Operator/1 -> Product/1
  Add1/1 -> Product/2
  Constant/1 -> Add1/1
  Reset/1 -> Logical Operator/1
  Memory/1 -> Add1/2

== system SUT_Test/Test Specification/R1 Speed Control step response/Maximum overshoot < 5 &  Steady state error < 5/Step response characteristics/Step response characteristics extraction/Extract maximum overshoot/Step response moving average and initial conditions before step/Flip if new step ==
  Enable : EnablePort
  Logical Operator : Logic  Operator=NOT  AllPortsSameDT=off  OutDataTypeMode=boolean
  Memory : Memory  Orientation=left
  0/1 : Outport  OutDataType=sfix(16)  OutScaling=2^0
  wires:
  Memory/1 -> Logical Operator/1
  Logical Operator/1 -> 0/1/1, Memory/1

== system SUT_Test/Test Specification/R1 Speed Control step response/Maximum overshoot < 5 &  Steady state error < 5/Step response characteristics/Step response characteristics extraction/Extract maximum overshoot/Trigger hold value/Negative step ==
  u : Inport  OutDataType=sfix(16)  OutScaling=2^0
  Compare : RelationalOperator  Operator=>  LogicOutDataTypeMode=Specify via dialog  ZeroCross=off  InputSameDT=on
  Ground : Ground
  y : Outport  OutDataType=sfix(16)  OutScaling=2^0
  wires:
  Compare/1 -> y/1
  Ground/1 -> Compare/2
  u/1 -> Compare/1

== system SUT_Test/Test Specification/R1 Speed Control step response/Maximum overshoot < 5 &  Steady state error < 5/Step response characteristics/Step response characteristics extraction/Extract maximum overshoot/Trigger hold value/Positive step ==
  u : Inport  OutDataType=sfix(16)  OutScaling=2^0
  Compare : RelationalOperator  Operator=<  LogicOutDataTypeMode=Specify via dialog  ZeroCross=off  InputSameDT=on
  Ground : Ground
  y : Outport  OutDataType=sfix(16)  OutScaling=2^0
  wires:
  Compare/1 -> y/1
  Ground/1 -> Compare/2
  u/1 -> Compare/1

== system SUT_Test/Test Specification/R1 Speed Control step response/Maximum overshoot < 5 &  Steady state error < 5/Step response characteristics/Step response characteristics extraction/Extract rise time/Time difference/Execution counter ==
  Reset : Inport  OutDataType=sfix(16)  OutScaling=2^0
  Add1 : Sum  OutDataType=sfix(16)  OutScaling=2^-10
  Constant : Constant  OutDataType=sfix(16)  OutScaling=2^0
  Logical Operator : Logic  Operator=NOT  AllPortsSameDT=off  OutDataTypeMode=Specify via dialog
  Memory : Memory  Orientation=left  InheritSampleTime=on
  Product : Product  OutDataType=sfix(16)  OutScaling=2^0  RndMeth=Zero
  Counter : Outport  OutDataType=sfix(16)  OutScaling=2^0
  wires:
  Product/1 -> Counter/1, Memory/1
  Logical Operator/1 -> Product/1
  Add1/1 -> Product/2
  Constant/1 -> Add1/1
  Reset/1 -> Logical Operator/1
  Memory/1 -> Add1/2

== system SUT_Test/Test Specification/R1 Speed Control step response/Maximum overshoot < 5 &  Steady state error < 5/Step response characteristics/Step response reset/Active if signals constant for some specified time/Time since signal constant/Detect constant ==
  Signal : Inport  OutDataType=sfix(16)  OutScaling=2^0
  Clock : Clock
      settings: Decimation=10
  Constant1 : Constant  Value=0  OutDataTypeMode=boolean  OutDataType=sfix(16)  OutScaling=2^0
  Memory : Memory
  Relative tolerance : Subsystem
  Switch : Switch  Criteria=u2 > Threshold
  Constant : Outport  OutDataType=sfix(16)  OutScaling=2^0
  wires:
  Signal/1 -> Memory/1, Relative tolerance/1(sig)
  Memory/1 -> Relative tolerance/2(ref)
  Constant1/1 -> Switch/3
  Clock/1 -> Switch/2
  Relative tolerance/1(sig == ref) -> Switch/1
  Switch/1 -> Constant/1

== system SUT_Test/Test Specification/R1 Speed Control step response/Maximum overshoot < 5 &  Steady state error < 5/Step response characteristics/Step response reset/Active if signals constant for some specified time/Time since signal constant1/Detect constant ==
  Signal : Inport  OutDataType=sfix(16)  OutScaling=2^0
  Clock : Clock
      settings: Decimation=10
  Constant1 : Constant  Value=0  OutDataTypeMode=boolean  OutDataType=sfix(16)  OutScaling=2^0
  Memory : Memory
  Relative tolerance : Subsystem
  Switch : Switch  Criteria=u2 > Threshold
  Constant : Outport  OutDataType=sfix(16)  OutScaling=2^0
  wires:
  Switch/1 -> Constant/1
  Relative tolerance/1(sig == ref) -> Switch/1
  Clock/1 -> Switch/2
  Constant1/1 -> Switch/3
  Memory/1 -> Relative tolerance/2(ref)
  Signal/1 -> Memory/1, Relative tolerance/1(sig)

== system SUT_Test/Test Specification/R1 Speed Control step response/Maximum overshoot < 5 &  Steady state error < 5/Step response characteristics/Step response trigger/Active if signals constant for some specified time/Time since signal constant/Detect constant ==
  Signal : Inport  OutDataType=sfix(16)  OutScaling=2^0
  Clock : Clock
      settings: Decimation=10
  Constant1 : Constant  Value=0  OutDataTypeMode=boolean  OutDataType=sfix(16)  OutScaling=2^0
  Memory : Memory
  Relative tolerance : Subsystem
  Switch : Switch  Criteria=u2 > Threshold
  Constant : Outport  OutDataType=sfix(16)  OutScaling=2^0
  wires:
  Signal/1 -> Memory/1, Relative tolerance/1(sig)
  Memory/1 -> Relative tolerance/2(ref)
  Constant1/1 -> Switch/3
  Clock/1 -> Switch/2
  Relative tolerance/1(sig == ref) -> Switch/1
  Switch/1 -> Constant/1

== system SUT_Test/Test Specification/R1 Speed Control step response/Maximum overshoot < 5 &  Steady state error < 5/Step response characteristics/Step response trigger/Active if signals constant for some specified time/Time since signal constant1/Detect constant ==
  Signal : Inport  OutDataType=sfix(16)  OutScaling=2^0
  Clock : Clock
      settings: Decimation=10
  Constant1 : Constant  Value=0  OutDataTypeMode=boolean  OutDataType=sfix(16)  OutScaling=2^0
  Memory : Memory
  Relative tolerance : Subsystem
  Switch : Switch  Criteria=u2 > Threshold
  Constant : Outport  OutDataType=sfix(16)  OutScaling=2^0
  wires:
  Switch/1 -> Constant/1
  Relative tolerance/1(sig == ref) -> Switch/1
  Clock/1 -> Switch/2
  Constant1/1 -> Switch/3
  Memory/1 -> Relative tolerance/2(ref)
  Signal/1 -> Memory/1, Relative tolerance/1(sig)

== system SUT_Test/Test Specification/R2 Speed Control velocity restoration time after simple  acceleration/deceleration/CC active + no target & Speed Control active & step of V_Des = |1|  with time periods >= 7s/Step with step size=|1|  and time periods >= 6s detection/Step detection/Active if signals constant for some specified time/Time since signal constant1/Detect constant ==
  Signal : Inport  OutDataType=sfix(16)  OutScaling=2^0
  Clock : Clock
      settings: Decimation=10
  Constant1 : Constant  Value=0  OutDataTypeMode=boolean  OutDataType=sfix(16)  OutScaling=2^0
  Memory : Memory
  Relative tolerance : Subsystem
  Switch : Switch  Criteria=u2 > Threshold
  Constant : Outport  OutDataType=sfix(16)  OutScaling=2^0
  wires:
  Switch/1 -> Constant/1
  Relative tolerance/1(sig == ref) -> Switch/1
  Clock/1 -> Switch/2
  Constant1/1 -> Switch/3
  Memory/1 -> Relative tolerance/2(ref)
  Signal/1 -> Memory/1, Relative tolerance/1(sig)

== system SUT_Test/Test Specification/R1 Speed Control step response/Complete step & CC active + no target & Speed Control active/Complete step detection/Step detection/Active if signals constant for some specified time/Time since signal constant/Detect constant/Relative tolerance ==
  sig : Inport  OutDataType=sfix(16)  OutScaling=2^0
  ref : Inport  Port=2  OutDataType=sfix(16)  OutScaling=2^0
  Abs : Abs
  Abs1 : Abs
  Add : Sum  Inputs=+-  OutDataType=sfix(16)  OutScaling=2^-10
  Divide1 : Product  Inputs=**/  OutDataType=sfix(16)  OutScaling=2^-10
  Max : Constant  Value=100  OutDataType=sfix(16)  OutScaling=2^0
  Relational Operator : RelationalOperator  Operator=<=  LogicOutDataTypeMode=boolean
  Relative Tolerance : Constant  Value=0.001  OutDataType=sfix(16)  OutScaling=2^0
  sig == ref : Outport  OutDataType=sfix(16)  OutScaling=2^0
  wires:
  Abs1/1 -> Divide1/1
  Relational Operator/1 -> sig == ref/1
  Relative Tolerance/1 -> Divide1/2
  Max/1 -> Divide1/3
  Divide1/1 -> Relational Operator/2
  ref/1 -> Abs1/1, Add/2
  sig/1 -> Add/1
  Add/1 -> Abs/1
  Abs/1 -> Relational Operator/1

== system SUT_Test/Test Specification/R1 Speed Control step response/Complete step & CC active + no target & Speed Control active/Complete step detection/Step detection/Active if signals constant for some specified time/Time since signal constant1/Detect constant/Relative tolerance ==
  sig : Inport  OutDataType=sfix(16)  OutScaling=2^0
  ref : Inport  Port=2  OutDataType=sfix(16)  OutScaling=2^0
  Abs : Abs
  Abs1 : Abs
  Add : Sum  Inputs=+-  OutDataType=sfix(16)  OutScaling=2^-10
  Divide1 : Product  Inputs=**/  OutDataType=sfix(16)  OutScaling=2^-10
  Max : Constant  Value=100  OutDataType=sfix(16)  OutScaling=2^0
  Relational Operator : RelationalOperator  Operator=<=  LogicOutDataTypeMode=boolean
  Relative Tolerance : Constant  Value=0.001  OutDataType=sfix(16)  OutScaling=2^0
  sig == ref : Outport  OutDataType=sfix(16)  OutScaling=2^0
  wires:
  Abs1/1 -> Divide1/1
  Relational Operator/1 -> sig == ref/1
  Relative Tolerance/1 -> Divide1/2
  Max/1 -> Divide1/3
  Divide1/1 -> Relational Operator/2
  ref/1 -> Abs1/1, Add/2
  sig/1 -> Add/1
  Add/1 -> Abs/1
  Abs/1 -> Relational Operator/1

== system SUT_Test/Test Specification/R1 Speed Control step response/Complete step & CC active + no target & Speed Control active/Complete step detection/Step detection reset/Active if signals constant for some specified time/Time since signal constant/Detect constant/Relative tolerance ==
  sig : Inport  OutDataType=sfix(16)  OutScaling=2^0
  ref : Inport  Port=2  OutDataType=sfix(16)  OutScaling=2^0
  Abs : Abs
  Abs1 : Abs
  Add : Sum  Inputs=+-  OutDataType=sfix(16)  OutScaling=2^-10
  Divide1 : Product  Inputs=**/  OutDataType=sfix(16)  OutScaling=2^-10
  Max : Constant  Value=100  OutDataType=sfix(16)  OutScaling=2^0
  Relational Operator : RelationalOperator  Operator=<=  LogicOutDataTypeMode=boolean
  Relative Tolerance : Constant  Value=0.0001  OutDataType=sfix(16)  OutScaling=2^0
  sig == ref : Outport  OutDataType=sfix(16)  OutScaling=2^0
  wires:
  Abs/1 -> Relational Operator/1
  Add/1 -> Abs/1
  sig/1 -> Add/1
  ref/1 -> Add/2, Abs1/1
  Divide1/1 -> Relational Operator/2
  Max/1 -> Divide1/3
  Relative Tolerance/1 -> Divide1/2
  Relational Operator/1 -> sig == ref/1
  Abs1/1 -> Divide1/1
